simulink model "inputtest"  (R2020b)
settings: Solver=VariableStepAuto  StartTime=0.0  StopTime=10  RelTol=1e-3
settings Model: Creator=Rick  LastModifiedBy=Rick

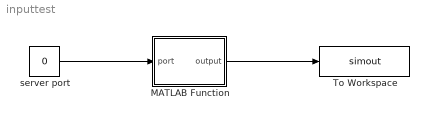
== system inputtest ==
  MATLAB Function : MATLAB Function  TreatAsAtomicUnit=on
  To Workspace : ToWorkspace  VariableName=simout  SaveFormat=Timeseries  SampleTime=-1
  server port : Constant  Value=0
  wires:
  MATLAB Function/1(output) -> To Workspace/1
  server port/1 -> MATLAB Function/1(port)

== matlab function inputtest/MATLAB Function ==
  data: output output; port input
function output = fcn(port)
    coder.extrinsic('tcpclient', 'write', 'readline');
    
    persistent client % use one client for one simulation
    if isempty(client)
        client = tcpclient('127.0.0.1', port, "Timeout", 10*60); % a minute long timeout just to be sure
    end
    
    write(client, "some message", "string");
    data = readline(client);
    
    output = 0;
    output = str2double(data);
